simulink model "WCS351571"  (R2019b)
settings: Solver=FixedStepAuto  StartTime=0.0  StopTime=10.0  FixedStep=0.01  RelTol=1e-3  EnableMultiTasking=on
settings Model: Creator=Alexander  LastModifiedBy=Alexander
settings OptimizationCC: DefaultParameterBehavior=Inlined  UseDivisionForNetSlopeComputation=on  EnhancedBackFolding=on  PassReuseOutputArgsAs=Individual arguments  ZeroExternalMemoryAtStartup=off  ZeroInternalMemoryAtStartup=off  EfficientFloat2IntCast=on  EfficientMapNaN2IntZero=off  MaxStackSize=inf  OptimizeBlockOrder=speed  DifferentSizesBufferReuse=on  OptimizationCustomize=off  EfficientTunableParamExpr=on
settings DebuggingCC: ReadBeforeWriteMsg=DisableAll  WriteAfterWriteMsg=DisableAll  WriteAfterReadMsg=DisableAll  MultiTaskDSMMsg=none  ParameterTunabilityLossMsg=error  AssertControl=DisableAll  SFUndirectedBroadcastEventsDiag=error
settings ModelReferenceCC: UpdateModelReferenceTargets=IfOutOfDate
settings SFSimCC: SFSimEcho=off  CompileTimeRecursionLimit=0  EnableRuntimeRecursion=off  MATLABDynamicMemAlloc=off
settings RTWCC: SystemTargetFile=ert.tlc  TemplateMakefile=ert_default_tmf  GenerateReport=on  IncludeHyperlinkInReport=on  LaunchReport=on  GenerateTraceInfo=on  GenerateTraceReport=on  GenerateTraceReportSl=on  GenerateTraceReportSf=on  GenerateTraceReportEml=on
settings CodeAppCC: ForceParamTrailComments=on  IgnoreCustomStorageClasses=off  OperatorAnnotations=on  SimulinkDataObjDesc=on  SFDataObjDesc=on  MATLABFcnDesc=on  InsertBlockDesc=on
settings ERTTargetCC: TargetLangStandard=C99 (ISO)  UtilityFuncGeneration=Shared location  GenerateSampleERTMain=on  IncludeMdlTerminateFcn=off  ParenthesesLevel=Maximum  CastingMode=Standards  GenerateSharedConstants=off  InlinedParameterPlacement=NonHierarchical  ERTCustomFileTemplate=example_file_process.tlc  PreserveIfCondition=on  EnableSignedLeftShifts=off  EnableSignedRightShifts=off

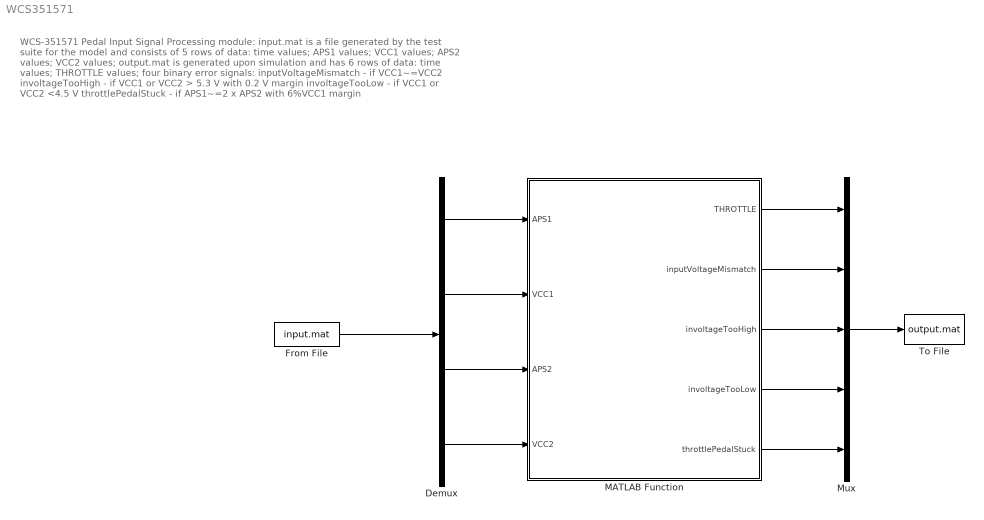
== system WCS351571 ==
  note: WCS-351571 Pedal Input Signal Processing module:
      |
      | input.mat is a file generated by the test suite for the model and consists of 5 rows of data:
      | time values;
      | APS1 values;
      | VCC1 values;
      | APS2 values;
      | VCC2 values;
      |
      | output.mat is generated upon simulation and has 6 rows of data:
      | time values;
      | THROTTLE values;
      | four binary error signals:
      | inputVoltageMismatch - if VCC1~=VCC2
      | involtageTooHigh - if VCC1 or VCC2 > 5.3 V with 0.2 V margin
      | involtageTooLow - if VCC1 or VCC2 <4.5 V
      | throttlePedalStuck - if APS1~=2 x APS2 with 6%VCC1 margin
  Demux : Demux
  From File : FromFile  FileName=input.mat  SampleTime=0.01
  MATLAB Function : MATLAB Function  TreatAsAtomicUnit=on
  Mux : Mux  Inputs=5
  To File : ToFile  Filename=output.mat  MatrixName=outputs  SampleTime=0.01
  wires:
  Demux/1 -> MATLAB Function/1(APS1)
  Demux/2 -> MATLAB Function/2(VCC1)
  Demux/3 -> MATLAB Function/3(APS2)
  Demux/4 -> MATLAB Function/4(VCC2)
  MATLAB Function/1(THROTTLE) -> Mux/1
  MATLAB Function/2(inputVoltageMismatch) -> Mux/2
  MATLAB Function/3(involtageTooHigh) -> Mux/3
  MATLAB Function/4(involtageTooLow) -> Mux/4
  MATLAB Function/5(throttlePedalStuck) -> Mux/5
  Mux/1 -> To File/1
  From File/1 -> Demux/1

== matlab function WCS351571/MATLAB Function ==
  data: APS1 input; THROTTLE output; VCC1 input; APS2 input; VCC2 input; inputVoltageMismatch output; involtageTooHigh output; involtageTooLow output; throttlePedalStuck output
function [THROTTLE,inputVoltageMismatch,...
      involtageTooHigh,involtageTooLow,throttlePedalStuck]= WCS351571(APS1, VCC1, APS2, VCC2)
%%
% Function inputs are two sensors signals: ARS1 and ARS2 in [V]:
%   APS1 is used for engine control,
%   APS2 is used for stuck pedal/throttle routine,
% and voltage power for the sensors in [V]:
%   VCC1 is APS1 sensor power,
%   VCC2 is APS2 sensor power.
%
% Function outputs are:
%   THROTTLE is pedal angular position in [%],
%   ERROR signals:
%       inputVoltageMismatch - if VCC1~=VCC2
%       throttlePedalStuck - if APS1~=2 x APS2 with 6%VCC1 margin
%       involtageTooHigh - if VCC1 or VCC2 > 5.3 V with 0.2 V margin
%       involtageTooLow - if VCC1 or VCC2 <4.5 V
%%

inputVoltageMismatch = 0;
involtageTooHigh = 0;
involtageTooLow = 0;
throttlePedalStuck = 0;

%%
if APS1<=0.22*VCC1                          % limit ARS1 to 22 - 84 %VCC1
    APS1=0.22*VCC1;
else
    if APS1>=0.84*VCC1
        APS1=0.84*VCC1;
    end
end
%%
if VCC1~=VCC2                               % check if VCC1 = VCC2
    inputVoltageMismatch = 1;
    THROTTLE=0;
else
    if VCC1>=5.3 || VCC2>=5.3
        involtageTooHigh = 1;
        THROTTLE=0;
    else
        if VCC1<=4.5 || VCC2<=4.5
            involtageTooLow = 1;
            THROTTLE=0;
        else
            if abs(APS1-2*APS2)/APS1>=0.06*VCC1      % check if ARS1 is twice ARS2 with 6%VCC1 margin
                throttlePedalStuck = 1;
                THROTTLE=0;
            else
                arsPerCent = (APS1/VCC1)*100;       % calculate ARS1 signal in percent of VCC1
                THROTTLE=round(1.613*arsPerCent-35.483);      % calculate THROTTLE signal is percent
            end
        end
    end
end
end
